simulink model "hgo_diff_with_plant2"  (R2024b)
settings: Solver=FixedStepAuto  StartTime=0.0  StopTime=15  FixedStep=1e-5  RelTol=1e-3
libraries: simulink x1, slpidlib x1
settings Model: Creator=user  LastModifiedBy=user

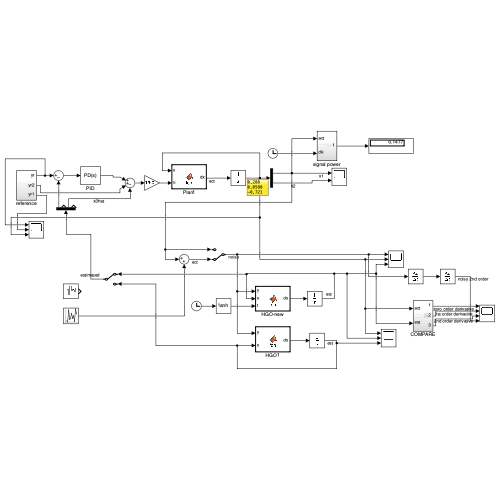
[thumbnail: Simulink's stored preview of the top-level diagram]
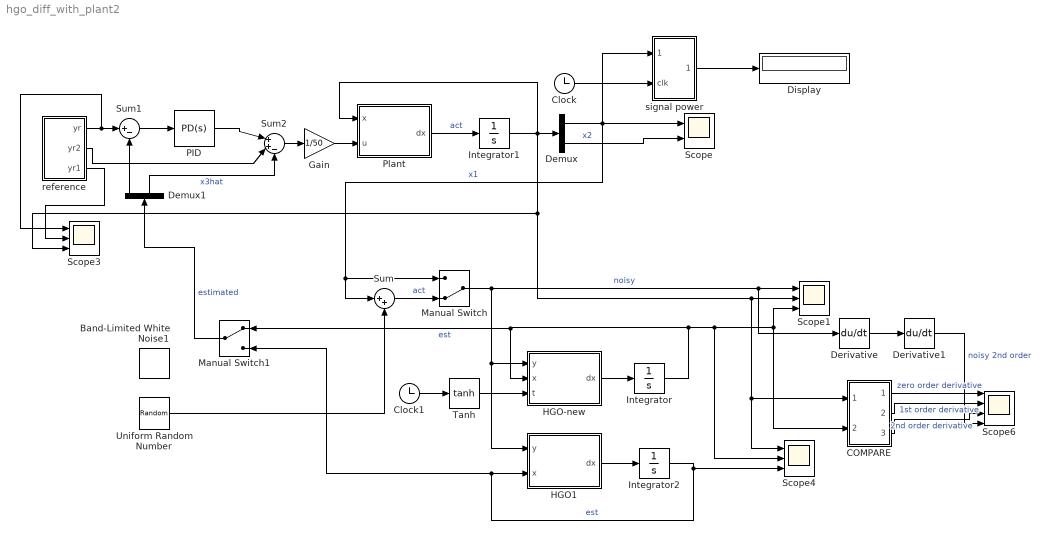
== system hgo_diff_with_plant2 ==
  Band-Limited White Noise1 : simulink/Sources/Band-Limited White Noise  Cov=1e-8  Ts=0.001  seed=[23341]
  COMPARE : Subsystem
  Clock : Clock
  Clock1 : Clock
  Demux : Demux  Outputs=[1 2]
  Demux1 : Demux
  Derivative : Derivative
  Derivative1 : Derivative
  Display : Display
  Gain : Gain  Gain=1/50
  HGO-new : MATLAB Function  TreatAsAtomicUnit=on
  HGO1 : MATLAB Function  TreatAsAtomicUnit=on
  Integrator : Integrator
  Integrator1 : Integrator
  Integrator2 : Integrator
  Manual Switch : ManualSwitch  CurrentSetting=0
  Manual Switch1 : ManualSwitch
  PID : slpidlib/PID Controller  Controller=PD  Form=Parallel  TimeDomain=Continuous-time  UseExternalTs=off  SampleTime=-1  IntegratorMethod=Forward Euler  FilterMethod=Forward Euler  ControllerParametersSource=internal  P=20  I=7.89124673404359e-08  UseKiTs=off  D=5  UseExternalDerivativeSource=off  N=100  UseFilter=on  TunerSelectOption=Transfer Function Based (PID Tuner App)  InitialConditionSource=internal  InitialConditionForIntegrator=0  InitialConditionForFilter=0  DifferentiatorICPrevScaledInput=0  ExternalReset=none  TrackingMode=off  Kt=1  LimitOutput=off  SatLimitsSource=internal  UpperSaturationLimit=inf  LowerSaturationLimit=-inf  LinearizeAsGain=on  AntiWindupMode=none  Kb=1  LimitIntegrator=off  UpperIntegratorSaturationLimit=inf  LowerIntegratorSaturationLimit=-inf  POutMin=[]  POutMax=[]  IOutMin=[]  IOutMax=[]  DOutMin=[]  DOutMax=[]  NOutMin=[]  NOutMax=[]  SumOutMin=[]  SumOutMax=[]  SaturationOutMin=[]  SaturationOutMax=[]  PParamMin=[]  PParamMax=[]  IParamMin=[]  IParamMax=[]  DParamMin=[]  DParamMax=[]  NParamMin=[]  NParamMax=[]  KbParamMin=[]  KbParamMax=[]  KtParamMin=[]  KtParamMax=[]  KbOutMin=[]  KbOutMax=[]  KtOutMin=[]  KtOutMax=[]  IntegratorOutMin=[]  IntegratorOutMax=[]  FilterOutMin=[]  FilterOutMax=[]  SumI1OutMin=[]  SumI1OutMax=[]  SumI2OutMin=[]  SumI2OutMax=[]  SumI3OutMin=[]  SumI3OutMax=[]  SumI4OutMin=[]  SumI4OutMax=[]  SumDOutMin=[]  SumDOutMax=[]  DifferentiatorOutMin=[]  DifferentiatorOutMax=[]  FilterDiffOutCoefMin=[]  FilterDiffOutCoefMax=[]  ReciprocalOutMin=[]  ReciprocalOutMax=[]  SumDenOutMin=[]  SumDenOutMax=[]  SumNumOutMin=[]  SumNumOutMax=[]  DivideOutMin=[]  DivideOutMax=[]  UdiffTsProdOutMin=[]  UdiffTsProdOutMax=[]  NTsProdOutMin=[]  NTsProdOutMax=[]  UintegralTsProdOutMin=[]  UintegralTsProdOutMax=[]  UngainTsProdOutMin=[]  UngainTsProdOutMax=[]  ClampingZeroOutDataTypeStr=Inherit: Inherit via back propagation  ClampingZeroOutMin=[]  ClampingZeroOutMax=[]  FilterDenConstantOutDataTypeStr=Inherit: Inherit via back propagation  FilterDenConstantOutMin=[]  FilterDenConstantOutMax=[]  PCopyOutDataTypeStr=Inherit: Inherit via back propagation  PCopyOutMin=[]  PCopyOutMax=[]  NCopyOutDataTypeStr=Inherit: Inherit via back propagation  NCopyOutMin=[]  NCopyOutMax=[]  IntegratorContinuousStateAttributes=''  IntegratorStateMustResolveToSignalObject=off  IntegratorRTWStateStorageClass=Auto  FilterContinuousStateAttributes=''  FilterStateMustResolveToSignalObject=off  FilterRTWStateStorageClass=Auto  ParallelPVariant=InternalParameters  IdealPVariant=Disabled  IVariant=Disabled  DVariant=InternalParameters  IntegratorVariant=Disabled  SatVariant=Disabled  AWVariant=Disabled  PCopyVariant=Disabled  TRVariant=Disabled  FdbkBlocksVariant=Forward  IdealPFdbkVariant=Disabled  SatFdbkVariant=Disabled  DerivativeFilterVariant=ContFilter  NVariant=InternalParameters  NCopyVariant=Disabled  FilterICVariant=InternalICsFilter  IntegratorICVariant=Disabled  ExternalResetVariant=Disabled  TRSumVariant=Passthrough  SumFdbkVariant=Disabled  SumVariant=Sum_PD  TsampFilterVariant=InternalTs  TsampNgainVariant=Passthrough  TsampIntegralVariant=Disabled_SignalSpec  ExternalSaturationOutDataTypeStr=Inherit: Same as second input  DerivativeSourceVariant=ErrorSignal  PreIntVariant=InternalPreInt
  Plant : MATLAB Function  TreatAsAtomicUnit=on
  Scope : Scope  NumInputPorts=2
  Scope1 : Scope  NumInputPorts=3
  Scope3 : Scope  NumInputPorts=3
  Scope4 : Scope  NumInputPorts=3
  Scope6 : Scope  NumInputPorts=4
  Sum : Sum  Inputs=|++
  Sum1 : Sum  Inputs=|+-
  Sum2 : Sum  Inputs=|++-
  Tanh : Trigonometry  Operator=tanh
  Uniform Random Number : UniformRandomNumber  Minimum=-1e-3  Maximum=1e-3  SampleTime=1e-3
  reference : Subsystem
  signal power : Subsystem
  wires:
  HGO-new/1(dx) -> Integrator/1
  Integrator/1 -> HGO-new/2(x), Manual Switch1/1, Scope4/2, Scope1/3, COMPARE/2(est)  "est"
  Sum/1 -> Manual Switch/2  "act"
  Manual Switch/1 -> Scope1/1, Derivative/1, HGO-new/1(y), HGO1/1(y)  "noisy"
  HGO1/1(dx) -> Integrator2/1
  Integrator2/1 -> Scope4/3, Manual Switch1/2, HGO1/2(x)  "est"
  Clock/1 -> signal power/2(clk)
  COMPARE/1(Out1) -> Scope6/1  "zero order derivative"
  COMPARE/2(Out2) -> Scope6/2  "1st order derivative"
  COMPARE/3(Out3) -> Scope6/3  "2nd order derivative"
  Integrator1/1 -> Demux/1, Scope1/2, COMPARE/1(act), Scope4/1, Scope3/3, Plant/1(x)
  Demux/2 -> Scope/2  "x2"
  Derivative/1 -> Derivative1/1
  Derivative1/1 -> Scope6/4  "noisy 2nd order"
  Tanh/1 -> HGO-new/3(t)
  Uniform Random Number/1 -> Sum/2
  signal power/1(Out1) -> Display/1
  Demux/1 -> Manual Switch/1, Sum/1, Scope/1, signal power/1(act)  "x1"
  Clock1/1 -> Tanh/1
  Plant/1(dx) -> Integrator1/1  "act"
  reference/1(yr) -> Scope3/1, Sum1/1
  Manual Switch1/1 -> Demux1/1  "estimated"
  Gain/1 -> Plant/2(u)
  Sum1/1 -> PID/1
  reference/2(yr2) -> Sum2/2
  PID/1 -> Sum2/1
  Sum2/1 -> Gain/1
  Demux1/3 -> Sum2/3  "x3hat"
  reference/3(yr1) -> Scope3/2
  Demux1/1 -> Sum1/2

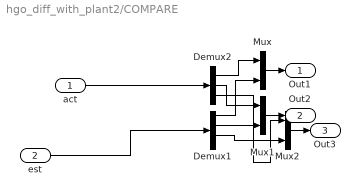
== system hgo_diff_with_plant2/COMPARE ==
  act : Inport
  est : Inport  Port=2
  Demux1 : Demux
  Demux2 : Demux  Outputs=3
  Mux : Mux  Inputs=2
  Mux1 : Mux  Inputs=2
  Mux2 : Mux  Inputs=2
  Out1 : Outport
  Out2 : Outport  Port=2
  Out3 : Outport  Port=3
  wires:
  est/1 -> Demux1/1
  Demux1/3 -> Mux2/2
  act/1 -> Demux2/1
  Demux2/1 -> Mux/1
  Mux/1 -> Out1/1
  Demux1/2 -> Mux1/2
  Demux1/1 -> Mux/2
  Demux2/2 -> Mux1/1
  Mux2/1 -> Out3/1
  Demux2/3 -> Mux2/1
  Mux1/1 -> Out2/1

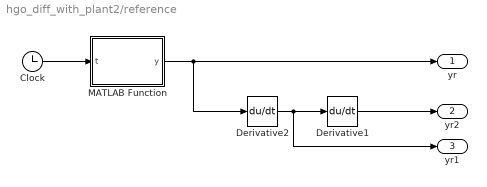
== system hgo_diff_with_plant2/reference ==
  Clock : Clock
  Derivative1 : Derivative
  Derivative2 : Derivative
  MATLAB Function : MATLAB Function  TreatAsAtomicUnit=on
  yr : Outport
  yr2 : Outport  Port=2
  yr1 : Outport  Port=3
  wires:
  Derivative2/1 -> yr1/1, Derivative1/1
  MATLAB Function/1(y) -> yr/1, Derivative2/1
  Derivative1/1 -> yr2/1
  Clock/1 -> MATLAB Function/1(t)

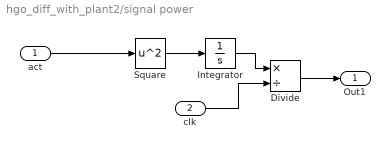
== system hgo_diff_with_plant2/signal power ==
  act : Inport
  clk : Inport  Port=2
  Divide : Product  Inputs=*/
  Integrator : Integrator
  Square : Math  Operator=square
  Out1 : Outport
  wires:
  Square/1 -> Integrator/1
  act/1 -> Square/1
  Integrator/1 -> Divide/1
  clk/1 -> Divide/2
  Divide/1 -> Out1/1

== matlab function hgo_diff_with_plant2/reference/MATLAB Function ==
  data: t input; y output
function y = fcn(t)

y = -cos(t)/(2+sin(3*t));

== matlab function hgo_diff_with_plant2/Plant ==
  data: x input; dx output; u input
function dx = fcn(x, u)
% x = [x1; x2; f]
Iy = 0.02; % moment
beta = 0.05; % drag coeff
dx = zeros(3,1);
A = [0 1 0;
      0 0 1;
      0 0 0];
B = [0; 0; 1/Iy];
F = [0; 0; 1/Iy];
C = [1; 0; 0];

dx = A*x + B*u - F*beta*x(2);

== matlab function hgo_diff_with_plant2/HGO-new ==
  data: y input; dx output; x input; t input
function dx = fcn(y, x, t)
    % Parameters
    n = 4;                % Order of the observer
    epsilon = 1/200;      % Small gain parameter
    tr = t/10; 
    % Binomial coefficients (for n = 4)
    % ki = nchoosek(n, i)
    k = [4, 6, 4, 1]; 

    e = 1e-5;
    % Initialize output derivative
    dx = zeros(n, 1);
    
    % High-Gain Observer Equations
    dx(1) = x(2) + (k(1)*(tr+e)^1 / epsilon^1) * (y - x(1));
    dx(2) = x(3) + (k(2)*(tr+e)^2 / epsilon^2) * (y - x(1));
    dx(3) = x(4) + (k(3)*(tr+e)^3 / epsilon^3) * (y - x(1));
    dx(4) = (k(4)*(tr+e)^4 / epsilon^4) * (y - x(1));
end

== matlab function hgo_diff_with_plant2/HGO1 ==
  data: y input; dx output; x input
function dx = fcn(y, x)
    % Parameters
    n = 4;                % Order of the observer
    epsilon = 1/150;      % Small gain parameter
    % tr = 1 ; 
    % Binomial coefficients (for n = 4)
    % ki = nchoosek(n, i)
    k = [4, 6, 4, 1]; 

    % Initialize output derivative
    dx = zeros(n, 1);
    
    % High-Gain Observer Equations
    dx(1) = x(2) + (k(1) / epsilon^1) * (y - x(1));
    dx(2) = x(3) + (k(2) / epsilon^2) * (y - x(1));
    dx(3) = x(4) + (k(3) / epsilon^3) * (y - x(1));
    dx(4) = (k(4) / epsilon^4) * (y - x(1));
end
